simulink model "vehicle_dynamics"  (Simulink 9.1)
settings: Solver=VariableStepAuto  StartTime=0.0  StopTime=10.0  RelTol=1e-3
model workspace (MAT data in the model file):
  map = Simulink.LookupTable
  map.Table = Simulink.lookuptable.Table
  map.Table.Dimensions = [0 0]
  map.Table.DataType = 'auto'
  map.Table.FieldName = 'Table'
  map.Breakpoints = Simulink.lookuptable.Breakpoint
  map.Breakpoints.TunableSizeName = 'N1'
  map.Breakpoints.Dimensions = [0 0]
  map.Breakpoints.DataType = 'auto'
  map.Breakpoints.FieldName = 'BP1'
  map.SupportTunableSize = 0
  map.StructTypeInfo = Simulink.lookuptable.StructTypeInfo
  map.StructTypeInfo.DataScope = 'Auto'
settings Model: Creator=Friends  LastModifiedBy=Friends
settings DataIOCC: SaveFormat=Dataset
settings OptimizationCC: LifeSpan=auto
settings DebuggingCC: UnderspecifiedInitializationDetection=Simplified  MergeDetectMultiDrivingBlocksExec=error  SFUnexpectedBacktrackingDiag=error  SFNoUnconditionalDefaultTransitionDiag=error  SFExecutionAtInitializationDiag=warning
settings HardwareCC: ProdBitPerPointer=64  ProdBitPerSizeT=64  ProdBitPerPtrDiffT=64  ProdLargestAtomicFloat=Float  ProdIntDivRoundTo=Zero  ProdEndianess=LittleEndian  ProdWordSize=64  ProdHWDeviceType=Intel->x86-64 (Windows64)
settings ModelReferenceCC: PropagateSignalLabelsOutOfModel=on
settings CodeAppCC: StateflowObjectComments=off
settings GRTTargetCC: TargetLangStandard=C99 (ISO)  CombineOutputUpdateFcns=on  GRTInterface=off
settings ConfigComp: CovMetricSettings=dwe  CovHtmlReporting=off  CovSaveCumulativeToWorkspaceVar=off  CovSaveSingleToWorkspaceVar=off  CovExternalEMLEnable=on

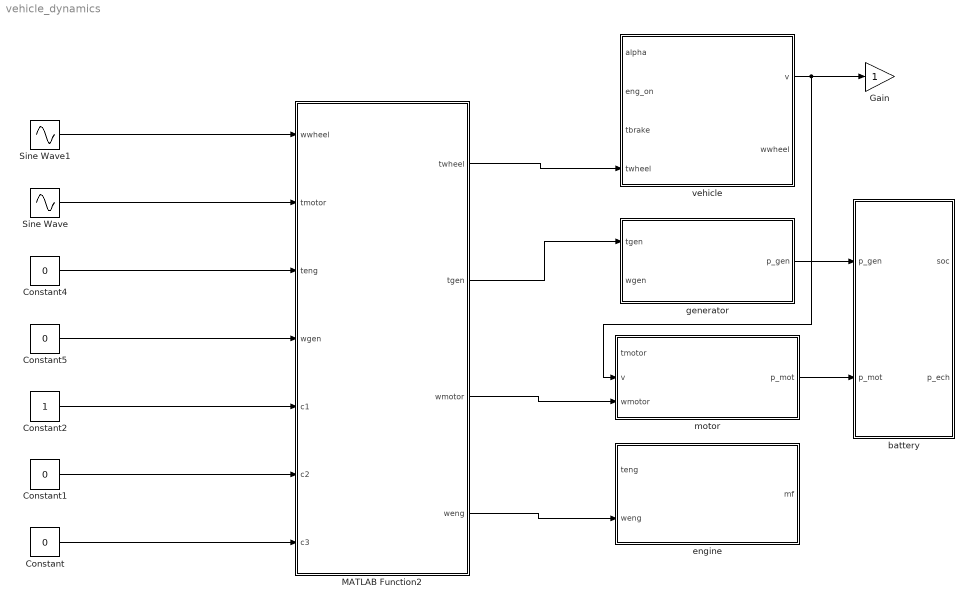
== system vehicle_dynamics ==
  Constant{,1,4..5} (4 alike) : Constant  Value=0
  Constant2 : Constant
  Gain : Gain
  MATLAB Function2 : MATLAB Function  TreatAsAtomicUnit=on
  Sine Wave : Sin  Amplitude=5  SampleTime=0
  Sine Wave1 : Sin  Amplitude=10  SampleTime=0
  battery : Subsystem
  engine : Subsystem
  generator : Subsystem
  motor : Subsystem
  vehicle : Subsystem
  wires:
  generator/1(p_gen) -> battery/1(p_gen)
  vehicle/1(v) -> motor/2(v), Gain/1
  motor/1(p_mot) -> battery/2(p_mot)
  Constant2/1 -> MATLAB Function2/5(c1)
  Constant1/1 -> MATLAB Function2/6(c2)
  Constant/1 -> MATLAB Function2/7(c3)
  Constant4/1 -> MATLAB Function2/3(teng)
  Constant5/1 -> MATLAB Function2/4(wgen)
  Sine Wave1/1 -> MATLAB Function2/1(wwheel)
  Sine Wave/1 -> MATLAB Function2/2(tmotor)
  MATLAB Function2/1(twheel) -> vehicle/4(twheel)
  MATLAB Function2/2(tgen) -> generator/1(tgen)
  MATLAB Function2/3(wmotor) -> motor/3(wmotor)
  MATLAB Function2/4(weng) -> engine/2(weng)

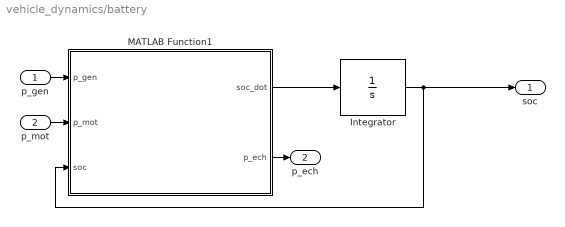
== system vehicle_dynamics/battery ==
  p_gen : Inport
  p_mot : Inport  Port=2
  Integrator : Integrator  InitialCondition=0.95
  MATLAB Function1 : MATLAB Function  TreatAsAtomicUnit=on
  soc : Outport
  p_ech : Outport  Port=2
  wires:
  MATLAB Function1/1(soc_dot) -> Integrator/1
  Integrator/1 -> soc/1, MATLAB Function1/3(soc)
  MATLAB Function1/2(p_ech) -> p_ech/1
  p_gen/1 -> MATLAB Function1/1(p_gen)
  p_mot/1 -> MATLAB Function1/2(p_mot)

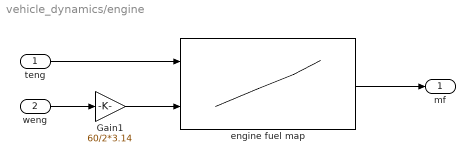
== system vehicle_dynamics/engine ==
  teng : Inport
  weng : Inport  Port=2
  Gain1 : Gain  Gain=60/2*3.14
  engine fuel map : Lookup_n-D  BreakpointsForDimension1=[0,10,20,30,40,50,60,70,80,90,100,110,120,130,140]  BreakpointsForDimension2=[1000,1500,2000,2500,3000,3500,4000,4500,5000]  BreakpointsForDimension3=[5, 7]  Table=reshape([0,0,0,0,0,0,0,0,0,0,0,0,0,0,0,0,0,400,330,300,280,270,260,250,250,250,0,0,0,0,0,0,400,330,300,280,270,260,250,240,240,250,0,0,0,0,0,400,330,300,280,270,250,250,250,240,240,240,0,0,0,0,400,330,300,280,270,250,250,240,240,250,250,0,0,0,0,400,330,300,280,270,260,260,260,260,260,260,260,0,0,0,400,400,300,280,270,270,270,270,270,270,270,270,0,0,0,400,400,400,330,300,300,300,300,300,300,300,300,0,0,0,0,0,0,0,0,0,0,0,0,0,0,0,0],15,9)  DiagnosticForOutOfRangeInput=Warning  InternalRulePriority=Speed  RndMeth=Simplest  InputSameDT=on
  mf : Outport
  wires:
  Gain1/1 -> engine fuel map/2
  engine fuel map/1 -> mf/1
  weng/1 -> Gain1/1
  teng/1 -> engine fuel map/1

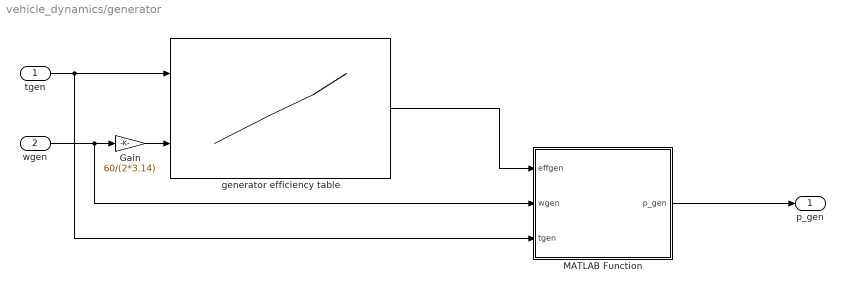
== system vehicle_dynamics/generator ==
  tgen : Inport
  wgen : Inport  Port=2
  Gain : Gain  Gain=60/(2*3.14)
  MATLAB Function : MATLAB Function  TreatAsAtomicUnit=on
  generator efficiency table : Lookup_n-D  BreakpointsForDimension1=[-200,-190,-180,-170,-160,-150,-140,-130,-120,-110,-100,-90,-80,-70,-60,-50,-40,-30,-20,-10,0]  BreakpointsForDimension2=[0,500,1000,1500,2000,2500,3000,3500,4000,4500,5000,5500,6000]  BreakpointsForDimension3=[5, 7]  Table=reshape([0,0,0,0,0,0,0,0,0,0,0,0,0,0,0,0,0,0,0,0,0,0,0,77,77,78,78,79,79,80,80,80,80,81,82,83,84,85,86,87,88,0,0,0,83,83,84,84,85,85,86,86,87,87,88,89,89,90,91,91,91,89,0,0,0,84,85,86,86,87,88,88,89,89,90,90,91,91,92,92,92,92,90,0,0,0,87,88,88,89,89,90,90,90,91,91,92,92,92,93,93,92,92,90,0,0,0,88,89,90,90,91,91,91,91,92,92,92,93,93,93,93,93,92,90,0,0,0,0,90,91,91,92,92,92,92,93,93,93,93,93,94,93,93,92,90,0,0,0,0,91,91,92,92,92,93,93,93,93,93,94,94,94,94,94,93,91,0,0,0,0,0,0,91,92,93,93,93,94,94,94,94,94,94,94,94,93,90,0,0,0,0,0,0,0,0,92,93,93,94,94,94,94,94,94,94,94,93,90,0,0,0,0,0,0,0,0,0,92,92,93,94,94,94,94,94,94,94,93,90,0,0,0,0,0,0,0,0,0,0,92,92,93,94,94,94,94,94,94,93,90,0,0,0,0,0,0,0,0,0,0,0,92,92,93,94,94,94,94,94,93,90,0],21,13)  DiagnosticForOutOfRangeInput=Warning  InternalRulePriority=Speed  RndMeth=Simplest  InputSameDT=on
  p_gen : Outport
  wires:
  generator efficiency table/1 -> MATLAB Function/1(effgen)
  MATLAB Function/1(p_gen) -> p_gen/1
  tgen/1 -> MATLAB Function/3(tgen), generator efficiency table/1
  wgen/1 -> Gain/1, MATLAB Function/2(wgen)
  Gain/1 -> generator efficiency table/2

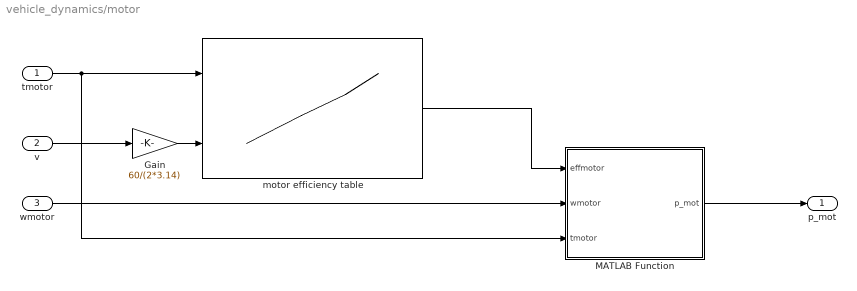
== system vehicle_dynamics/motor ==
  "tmotor " : Inport
  v : Inport  Port=2
  wmotor : Inport  Port=3
  Gain : Gain  Gain=60/(2*3.14)
  MATLAB Function : MATLAB Function  TreatAsAtomicUnit=on
  motor efficiency table : Lookup_n-D  BreakpointsForDimension1=[0,250,500,750,1000,1250,1500,1750,2000,2250,2500]  BreakpointsForDimension2=[0,25,50,75,100,125,150,175]  BreakpointsForDimension3=[5, 7]  Table=reshape([69,69,69,69,69,69,69,69,69,69,69,69,70,80,80,80,80,80,80,80,80,80,69,80,84,84,84,84,84,84,84,84,84,69,80,86,88,88,86,86,84,0,0,0,69,80,84,86,86,84,80,0,0,0,0,69,70,80,84,80,0,0,0,0,0,0,69,70,70,70,0,0,0,0,0,0,0,69,70,70,70,0,0,0,0,0,0,0],11,8)  DiagnosticForOutOfRangeInput=Warning  InternalRulePriority=Speed  RndMeth=Simplest  InputSameDT=on
  p_mot : Outport
  wires:
  wmotor/1 -> MATLAB Function/2(wmotor)
  "tmotor "/1 -> MATLAB Function/3(tmotor), motor efficiency table/1
  motor efficiency table/1 -> MATLAB Function/1(effmotor)
  v/1 -> Gain/1
  Gain/1 -> motor efficiency table/2
  MATLAB Function/1(p_mot) -> p_mot/1

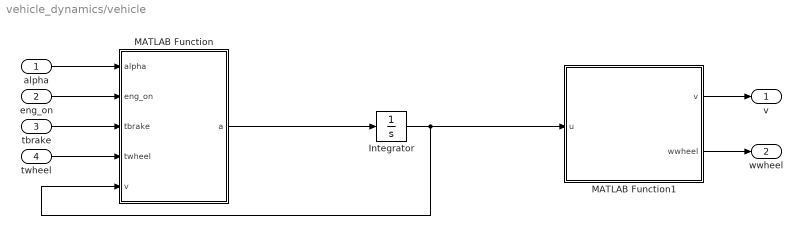
== system vehicle_dynamics/vehicle ==
  alpha : Inport
  eng_on : Inport  Port=2
  tbrake : Inport  Port=3
  twheel : Inport  Port=4
  Integrator : Integrator
  MATLAB Function : MATLAB Function  TreatAsAtomicUnit=on
  MATLAB Function1 : MATLAB Function  TreatAsAtomicUnit=on
  v : Outport
  wwheel : Outport  Port=2
  wires:
  MATLAB Function1/2(wwheel) -> wwheel/1
  Integrator/1 -> MATLAB Function/5(v), MATLAB Function1/1(u)
  twheel/1 -> MATLAB Function/4(twheel)
  MATLAB Function/1(a) -> Integrator/1
  eng_on/1 -> MATLAB Function/2(eng_on)
  MATLAB Function1/1(v) -> v/1
  tbrake/1 -> MATLAB Function/3(tbrake)
  alpha/1 -> MATLAB Function/1(alpha)

== matlab function vehicle/MATLAB Function1 ==
  data: u input double; v output double; wwheel output double
function [v,wwheel] = f(u)
r_wh = 33e-2; %m
wwheel = u/r_wh;
v = u;

== matlab function vehicle/MATLAB Function ==
  data: alpha input double; a output double; eng_on input double; tbrake input double; twheel input double; v input double
function a = v_dot(alpha, eng_on, tbrake, twheel, v)
    r_wh = 33e-2; %m
    c0 = 105.95; %N
    c1 = 0.01; %Ns/m
    c2 = 0.4340; %Ns^2/m^2
    Jv = 207; %kg m^2
    wb = 2685e-3; %m
    cogh = 550e-3;%m
    g = 9.81; %m/s^2
    mv = 1812; %kg
    
a =eng_on*((r_wh/Jv)*(tbrake + twheel - mv*r_wh*g*sin(deg2rad(alpha)) - r_wh*(c0 + c1*v + c2*v*v)));

== matlab function MATLAB Function2 ==
  data: twheel output double; tgen output double; wwheel input double; tmotor input double; teng input double; wgen input double; c1 input double; c2 input double; c3 input double; wmotor output double; weng output double
function [twheel,tgen,wmotor,weng] = powertrain(wwheel,tmotor,teng,wgen,c1,c2,c3)
rho=2.24; %nring/nsun
Rd=2.16; %differential gear ratio
% torques in Nm, angular speeds in rad/s
if (c1==1)&&(c2==0)&&(c3==0)
    tgen=0;
    twheel=Rd*(rho+1)*tmotor;
    weng=0;
    wmotor=wwheel*Rd*(rho+1);   
elseif (c1==0)&&(c2==1)&&(c3==0)
    tgen=rho*tmotor;
    twheel=Rd*(rho+1)*tmotor;
    weng=0;
    wmotor=wwheel*Rd*(rho+1)-wgen*rho;
elseif (c1==1)&&(c2==0)&&(c3==1)
    tgen=-teng;
    twheel=Rd*(rho+1)*tmotor;
    weng=wgen;
    wmotor=wwheel*Rd*(rho+1);
elseif (c1==0)&&(c2==1)&&(c3==1)
    tgen=rho*tmotor-teng;
    twheel=Rd*(rho+1)*tmotor;
    weng=wgen;
    wmotor=wwheel*Rd*(rho+1)-rho*wgen;
else
    tgen=0;
    twheel=0;
    weng=0;
    wmotor=0;
end

== matlab function generator/MATLAB Function ==
  data: effgen input double; p_gen output double; wgen input double; tgen input double
function p_gen = genpower(effgen,wgen,tgen)

p_gen = effgen*wgen*tgen;

== matlab function battery/MATLAB Function1 ==
  data: p_gen input double; soc_dot output double; p_mot input double; soc input double; p_ech output double
function [soc_dot, p_ech] = soc_dot(p_gen,p_mot,soc)
n_c=1;
Voc = 360; %volts
Q = 16000/360; %Ah
Ro = 100; %ohms, random value
P_bat = p_gen+p_mot;
I_bat = (Voc-sqrt(Voc^2 - 4*P_bat*Ro/soc))/(2*Ro);
p_ech = Voc*I_bat;
soc_dot = -n_c*I_bat/Q;

== matlab function motor/MATLAB Function ==
  data: effmotor input double; p_mot output double; wmotor input double; tmotor input double
function p_mot = motpower(effmotor,wmotor,tmotor)

p_mot = effmotor*wmotor*tmotor;
